simulink model "LLC_26"  (R2022b)
settings: Solver=VariableStepAuto  StartTime=0.0  StopTime=.01  RelTol=1e-3
values from neighbouring files (symbols this model uses):
  tsample_Controller = 20e-6    (= 2e-05)    [LLC_Parameter.m]
  Vref = 500    [LLC_Parameter.m]
undefined symbols (not defined in the file or in its folder): Iref
libraries: fl_lib x137, ee_lib x83, nesl_utility x63, slpidlib x7, slctrlblks x1
(part 5 of 5)

== system LLC_26/Subsystem5 ==
  Capacitor : ee_lib/Passive/Capacitor  cap_option=0  c=10e-6 F  Cvec=[1e-05, 1e-06] F  Vvec=[0, 10] V  CV_table_symmetry=1  f_vec=[1, 10] kHz  DFext_vec=[.8, 1.2]  enable_C_tol=0  C_tol=5  tol_distribution=1  nSigma=4  r=1e-6 Ohm  g=0 1/Ohm  averaging_period=0 s  enable_operating_limits=0  operating_limit_action=2  max_working_voltage_range=[-25, 25] V  power_rating=1 W  enable_faults=0  fault_action=1  Cscale_faulted=100  R_faulted=1e-3 Ohm  G_faulted=0 1/Ohm  tau_fault=1e-3 s  enable_temporal_fault=0  t_fault=1 s  enable_behavioral_fault=0  max_permissible_voltage_range=[-100, 100] V  t_fail_on_voltage=1 s  i_specify=off  i_priority=None  i=0 A  i_nominal_specify=off  i_nominal_unit=A  i_nominal_value=1  v_specify=off  v_priority=None  v=0 V  v_nominal_specify=off  v_nominal_unit=V  v_nominal_value=1  vc_specify=off  vc_priority=High  vc=0 V  vc_nominal_specify=off  vc_nominal_unit=V  vc_nominal_value=1
  Da{34..35,43..44} (4 alike) : ee_lib/Semiconductors & Converters/Diode  ModelType=ee.enum.diode.modelType.pwl  TableType=ee.enum.diode.tableType.IfMat  IfMat=[.07, .12, .19, 1.75, 4.24, 7.32, 11.2; .16, .3, .72, 2.14, 4.02, 6.35, 9.12] A  VfMat=[.9, 1.15, 1.25, 1.5, 1.75, 2.17, 2.6, 2.85; .58, .68, .75, 1.1, 1.38, 1.77, 2.27, 2.7] V  TjVec=[25, 125] degC  VfVec=[.5, .7, .9, 1.3, 1.7, 2.1, 2.5] V  IfVec=[.1, .2, .5, 1, 2, 4, 7, 10] A  Vf=Vf V  Ron=Ron Ohm  Goff=1e-8 1/Ohm  prmExp=ee.enum.diode.expParam.useTwo  I12=[.0137, .545] A  V12=[.6, .7] V  RS=0 Ohm  Tmeas=25 degC  IS=1e-12 A  ec=1  I1=0.0137 A  V1=0.6 V  N_series=1  N_parallel=1  Rz=0.3 Ohm  BV=inf V  C_param=ee.enum.diode.capParam.fixed  CJ=0 pF  CJ0=5 pF  Vvec=[.1, 10, 100] V  Cvec=[3.5, 1, .4] pF  VJ=1 V  Mgrad=0.5  FC=0.5  Q_param=ee.enum.diode.recoveryParam.off  iRM=-7.15 A  iF=4 A  didt=-750 A/us  trr_factor=3  trr=115 ns  Qrr=1500 s*uA  Vr=-600 V  Ls=150 nH  Erec=0.03 J  TT=50 ns  tau=100 ns  T_param=ee.enum.diode.temperatureParam.off  Tdevice=25 degC  I1_T2=0.245 A  V1_T2=0.5 V  IS_T2=1.25e-7 A  Tmeas2=125 degC  XTI_param=ee.enum.diode.xtiParam.pn  XTI=3  EG_param=ee.enum.diode.egapParam.material_si  EG=1.11 eV  dBVdT=0 V/K  enable_faults=simscape.enum.onoff.off  fault_action=simscape.enum.assert.action.none  fault_types=ee.enum.diode.faults.open  tau_fault=1e-3 s  IfMat_faulted=[.07, .12, .19, 1.75, 4.24, 7.32, 11.2; .16, .3, .72, 2.14, 4.02, 6.35, 9.12] A  VfMat_faulted=[.9, 1.15, 1.25, 1.5, 1.75, 2.17, 2.6, 2.85; .58, .68, .75, 1.1, 1.38, 1.77, 2.27, 2.7] V  VfVec_faulted=[.5, .7, .9, 1.3, 1.7, 2.1, 2.5] V  IfVec_faulted=[.1, .2, .5, 1, 2, 4, 7, 10] A  Ropen_faulted=1000 Ohm  Gshort_faulted=1000 1/Ohm  Vf_faulted=0.6 V  Ron_faulted=0.3 Ohm  Goff_faulted=1e-8 S  I12_faulted=[.0137, .545] A  V12_faulted=[.6, .7] V  IS_faulted=1e-12 A  ec_faulted=1  I1_faulted=0.0137 A  V1_faulted=0.6 V  RS_faulted=0 Ohm  Rz_faulted=0.3 Ohm  BV_faulted=inf V  Cscale_faulted=100  enable_temporal_fault=simscape.enum.onoff.off  t_fault=inf s  enable_behavioral_fault=simscape.enum.onoff.off  max_permissible_voltage=inf V  n_fail_on_voltage=1  max_permissible_current=inf A  t_fail_on_current=1 s  max_permissible_dVdt=inf V/s  enable_fault_input=simscape.enum.onoff.off  i_specify=off  i_priority=None  i=0 A  i_nominal_specify=off  i_nominal_unit=A  i_nominal_value=1  v_specify=off  v_priority=None  v=0 V  v_nominal_specify=off  v_nominal_unit=V  v_nominal_value=1  v_capacitor_specify=off  v_capacitor_priority=None  v_capacitor=0 V  v_capacitor_nominal_specify=off  v_capacitor_nominal_unit=V  v_capacitor_nominal_value=1  i_diode_specify=off  i_diode_priority=None  i_diode=0 A  i_diode_nominal_specify=off  i_diode_nominal_unit=A  i_diode_nominal_value=1  v_diode_specify=off  v_diode_priority=None  v_diode=0 V  v_diode_nominal_specify=off  v_diode_nominal_unit=V  v_diode_nominal_value=1  i_capacitor_specify=off  i_capacitor_priority=None  i_capacitor=0 A  i_capacitor_nominal_specify=off  i_capacitor_nominal_unit=A  i_capacitor_nominal_value=1  power_dissipated_specify=off  power_dissipated_priority=None  power_dissipated=0 W  power_dissipated_nominal_specify=off  power_dissipated_nominal_unit=W  power_dissipated_nominal_value=1  fidelity_level=ee.enum.diode.fidelity.includeChargeDyn  rec_loss_model=ee.enum.diode.reverseRecoveryModel.fixed  ErecVal=0 J  ErecMat=zeros(2, 3) J  TjrecVec=[298.15, 398.15] K  IfrecVec=[.1, 1, 10] A  VrecVal=10 V  tFilter=1 / 1000 / 100 s  max_permissible_temperature=inf K  t_fail_on_temperature=1 s  thermal_network_parameterization=ee.enum.thermalNetworkTopology.junctionCase  Rth=[0, 10] K/W  Rth_Cauer=[1, 3, 10] K/W  Rth_Foster=[4, 6] K/W  thermal_mass_parameterization=ee.enum.thermalNetwork.timeconstant  thermal_mass=[0, 1] J/K  thermal_mass_Cauer=[.1, .3, 1] J/K  thermal_mass_Foster=[1.5, 3] J/K  thermal_time_constant=[0, 10] s  thermal_time_constant_Cauer=[1, 3, 10] s  thermal_time_constant_Foster=[6, 18] s  thermal_mass_initial_temperatures=[25, 25] degC  thermal_mass_initial_temperatures_Cauer=[25, 25, 25] degC  junction_thermal_mass=0.01 J/K  Tvec_initial_Foster=[25, 25, 25, 25] degC  no_thermal_network=0  junction_temperature_specify=off  junction_temperature_priority=None  junction_temperature=25 degC  junction_temperature_nominal_specify=off  junction_temperature_nominal_unit=degC  junction_temperature_nominal_value=1
  Ph : PMIOPort  Side=Left
  N : PMIOPort  Port=2  Side=Left
  DC+ : PMIOPort  Port=3  Side=Right
  DC- : PMIOPort  Port=4  Side=Right
  connections:
  Da35/RConn1 -- Da43/LConn1 -- N/RConn1
  Da34/RConn1 -- Da44/LConn1 -- Ph/RConn1
  Da34/LConn1 -- Capacitor/RConn1 -- DC-/RConn1 -- Da35/LConn1
  DC+/RConn1 -- Da44/RConn1 -- Da43/RConn1 -- Capacitor/LConn1

== system LLC_26/Subsystem6 ==
  Capacitor : ee_lib/Passive/Capacitor  cap_option=0  c=10e-6 F  Cvec=[1e-05, 1e-06] F  Vvec=[0, 10] V  CV_table_symmetry=1  f_vec=[1, 10] kHz  DFext_vec=[.8, 1.2]  enable_C_tol=0  C_tol=5  tol_distribution=1  nSigma=4  r=1e-6 Ohm  g=0 1/Ohm  averaging_period=0 s  enable_operating_limits=0  operating_limit_action=2  max_working_voltage_range=[-25, 25] V  power_rating=1 W  enable_faults=0  fault_action=1  Cscale_faulted=100  R_faulted=1e-3 Ohm  G_faulted=0 1/Ohm  tau_fault=1e-3 s  enable_temporal_fault=0  t_fault=1 s  enable_behavioral_fault=0  max_permissible_voltage_range=[-100, 100] V  t_fail_on_voltage=1 s  i_specify=off  i_priority=None  i=0 A  i_nominal_specify=off  i_nominal_unit=A  i_nominal_value=1  v_specify=off  v_priority=None  v=0 V  v_nominal_specify=off  v_nominal_unit=V  v_nominal_value=1  vc_specify=off  vc_priority=High  vc=0 V  vc_nominal_specify=off  vc_nominal_unit=V  vc_nominal_value=1
  Capacitor1 : ee_lib/Passive/Capacitor  cap_option=0  c=10e-6 F  Cvec=[1e-05, 1e-06] F  Vvec=[0, 10] V  CV_table_symmetry=1  f_vec=[1, 10] kHz  DFext_vec=[.8, 1.2]  enable_C_tol=0  C_tol=5  tol_distribution=1  nSigma=4  r=1e-6 Ohm  g=0 1/Ohm  averaging_period=0 s  enable_operating_limits=0  operating_limit_action=2  max_working_voltage_range=[-25, 25] V  power_rating=1 W  enable_faults=0  fault_action=1  Cscale_faulted=100  R_faulted=1e-3 Ohm  G_faulted=0 1/Ohm  tau_fault=1e-3 s  enable_temporal_fault=0  t_fault=1 s  enable_behavioral_fault=0  max_permissible_voltage_range=[-100, 100] V  t_fail_on_voltage=1 s  i_specify=off  i_priority=None  i=0 A  i_nominal_specify=off  i_nominal_unit=A  i_nominal_value=1  v_specify=off  v_priority=None  v=0 V  v_nominal_specify=off  v_nominal_unit=V  v_nominal_value=1  vc_specify=off  vc_priority=High  vc=0 V  vc_nominal_specify=off  vc_nominal_unit=V  vc_nominal_value=1
  Da{34..35,43..44} (4 alike) : ee_lib/Semiconductors & Converters/Diode  ModelType=ee.enum.diode.modelType.pwl  TableType=ee.enum.diode.tableType.IfMat  IfMat=[.07, .12, .19, 1.75, 4.24, 7.32, 11.2; .16, .3, .72, 2.14, 4.02, 6.35, 9.12] A  VfMat=[.9, 1.15, 1.25, 1.5, 1.75, 2.17, 2.6, 2.85; .58, .68, .75, 1.1, 1.38, 1.77, 2.27, 2.7] V  TjVec=[25, 125] degC  VfVec=[.5, .7, .9, 1.3, 1.7, 2.1, 2.5] V  IfVec=[.1, .2, .5, 1, 2, 4, 7, 10] A  Vf=Vf V  Ron=Ron Ohm  Goff=1e-8 1/Ohm  prmExp=ee.enum.diode.expParam.useTwo  I12=[.0137, .545] A  V12=[.6, .7] V  RS=0 Ohm  Tmeas=25 degC  IS=1e-12 A  ec=1  I1=0.0137 A  V1=0.6 V  N_series=1  N_parallel=1  Rz=0.3 Ohm  BV=inf V  C_param=ee.enum.diode.capParam.fixed  CJ=0 pF  CJ0=5 pF  Vvec=[.1, 10, 100] V  Cvec=[3.5, 1, .4] pF  VJ=1 V  Mgrad=0.5  FC=0.5  Q_param=ee.enum.diode.recoveryParam.off  iRM=-7.15 A  iF=4 A  didt=-750 A/us  trr_factor=3  trr=115 ns  Qrr=1500 s*uA  Vr=-600 V  Ls=150 nH  Erec=0.03 J  TT=50 ns  tau=100 ns  T_param=ee.enum.diode.temperatureParam.off  Tdevice=25 degC  I1_T2=0.245 A  V1_T2=0.5 V  IS_T2=1.25e-7 A  Tmeas2=125 degC  XTI_param=ee.enum.diode.xtiParam.pn  XTI=3  EG_param=ee.enum.diode.egapParam.material_si  EG=1.11 eV  dBVdT=0 V/K  enable_faults=simscape.enum.onoff.off  fault_action=simscape.enum.assert.action.none  fault_types=ee.enum.diode.faults.open  tau_fault=1e-3 s  IfMat_faulted=[.07, .12, .19, 1.75, 4.24, 7.32, 11.2; .16, .3, .72, 2.14, 4.02, 6.35, 9.12] A  VfMat_faulted=[.9, 1.15, 1.25, 1.5, 1.75, 2.17, 2.6, 2.85; .58, .68, .75, 1.1, 1.38, 1.77, 2.27, 2.7] V  VfVec_faulted=[.5, .7, .9, 1.3, 1.7, 2.1, 2.5] V  IfVec_faulted=[.1, .2, .5, 1, 2, 4, 7, 10] A  Ropen_faulted=1000 Ohm  Gshort_faulted=1000 1/Ohm  Vf_faulted=0.6 V  Ron_faulted=0.3 Ohm  Goff_faulted=1e-8 S  I12_faulted=[.0137, .545] A  V12_faulted=[.6, .7] V  IS_faulted=1e-12 A  ec_faulted=1  I1_faulted=0.0137 A  V1_faulted=0.6 V  RS_faulted=0 Ohm  Rz_faulted=0.3 Ohm  BV_faulted=inf V  Cscale_faulted=100  enable_temporal_fault=simscape.enum.onoff.off  t_fault=inf s  enable_behavioral_fault=simscape.enum.onoff.off  max_permissible_voltage=inf V  n_fail_on_voltage=1  max_permissible_current=inf A  t_fail_on_current=1 s  max_permissible_dVdt=inf V/s  enable_fault_input=simscape.enum.onoff.off  i_specify=off  i_priority=None  i=0 A  i_nominal_specify=off  i_nominal_unit=A  i_nominal_value=1  v_specify=off  v_priority=None  v=0 V  v_nominal_specify=off  v_nominal_unit=V  v_nominal_value=1  v_capacitor_specify=off  v_capacitor_priority=None  v_capacitor=0 V  v_capacitor_nominal_specify=off  v_capacitor_nominal_unit=V  v_capacitor_nominal_value=1  i_diode_specify=off  i_diode_priority=None  i_diode=0 A  i_diode_nominal_specify=off  i_diode_nominal_unit=A  i_diode_nominal_value=1  v_diode_specify=off  v_diode_priority=None  v_diode=0 V  v_diode_nominal_specify=off  v_diode_nominal_unit=V  v_diode_nominal_value=1  i_capacitor_specify=off  i_capacitor_priority=None  i_capacitor=0 A  i_capacitor_nominal_specify=off  i_capacitor_nominal_unit=A  i_capacitor_nominal_value=1  power_dissipated_specify=off  power_dissipated_priority=None  power_dissipated=0 W  power_dissipated_nominal_specify=off  power_dissipated_nominal_unit=W  power_dissipated_nominal_value=1  fidelity_level=ee.enum.diode.fidelity.includeChargeDyn  rec_loss_model=ee.enum.diode.reverseRecoveryModel.fixed  ErecVal=0 J  ErecMat=zeros(2, 3) J  TjrecVec=[298.15, 398.15] K  IfrecVec=[.1, 1, 10] A  VrecVal=10 V  tFilter=1 / 1000 / 100 s  max_permissible_temperature=inf K  t_fail_on_temperature=1 s  thermal_network_parameterization=ee.enum.thermalNetworkTopology.junctionCase  Rth=[0, 10] K/W  Rth_Cauer=[1, 3, 10] K/W  Rth_Foster=[4, 6] K/W  thermal_mass_parameterization=ee.enum.thermalNetwork.timeconstant  thermal_mass=[0, 1] J/K  thermal_mass_Cauer=[.1, .3, 1] J/K  thermal_mass_Foster=[1.5, 3] J/K  thermal_time_constant=[0, 10] s  thermal_time_constant_Cauer=[1, 3, 10] s  thermal_time_constant_Foster=[6, 18] s  thermal_mass_initial_temperatures=[25, 25] degC  thermal_mass_initial_temperatures_Cauer=[25, 25, 25] degC  junction_thermal_mass=0.01 J/K  Tvec_initial_Foster=[25, 25, 25, 25] degC  no_thermal_network=0  junction_temperature_specify=off  junction_temperature_priority=None  junction_temperature=25 degC  junction_temperature_nominal_specify=off  junction_temperature_nominal_unit=degC  junction_temperature_nominal_value=1
  Ph : PMIOPort  Side=Left
  N : PMIOPort  Port=2  Side=Left
  DC+ : PMIOPort  Port=3  Side=Right
  DC- : PMIOPort  Port=4  Side=Right
  connections:
  Da35/RConn1 -- Da43/LConn1 -- N/RConn1
  Da34/RConn1 -- Da44/LConn1 -- Ph/RConn1
  Da34/LConn1 -- Capacitor/RConn1 -- DC-/RConn1 -- Capacitor1/RConn1 -- Da35/LConn1
  DC+/RConn1 -- Capacitor1/LConn1 -- Da44/RConn1 -- Da43/RConn1 -- Capacitor/LConn1

== system LLC_26/Subsystem7 ==
  Capacitor : ee_lib/Passive/Capacitor  cap_option=0  c=10e-6 F  Cvec=[1e-05, 1e-06] F  Vvec=[0, 10] V  CV_table_symmetry=1  f_vec=[1, 10] kHz  DFext_vec=[.8, 1.2]  enable_C_tol=0  C_tol=5  tol_distribution=1  nSigma=4  r=1e-6 Ohm  g=0 1/Ohm  averaging_period=0 s  enable_operating_limits=0  operating_limit_action=2  max_working_voltage_range=[-25, 25] V  power_rating=1 W  enable_faults=0  fault_action=1  Cscale_faulted=100  R_faulted=1e-3 Ohm  G_faulted=0 1/Ohm  tau_fault=1e-3 s  enable_temporal_fault=0  t_fault=1 s  enable_behavioral_fault=0  max_permissible_voltage_range=[-100, 100] V  t_fail_on_voltage=1 s  i_specify=off  i_priority=None  i=0 A  i_nominal_specify=off  i_nominal_unit=A  i_nominal_value=1  v_specify=off  v_priority=None  v=0 V  v_nominal_specify=off  v_nominal_unit=V  v_nominal_value=1  vc_specify=off  vc_priority=High  vc=0 V  vc_nominal_specify=off  vc_nominal_unit=V  vc_nominal_value=1
  Da{34..35,43..44} (4 alike) : ee_lib/Semiconductors & Converters/Diode  ModelType=ee.enum.diode.modelType.pwl  TableType=ee.enum.diode.tableType.IfMat  IfMat=[.07, .12, .19, 1.75, 4.24, 7.32, 11.2; .16, .3, .72, 2.14, 4.02, 6.35, 9.12] A  VfMat=[.9, 1.15, 1.25, 1.5, 1.75, 2.17, 2.6, 2.85; .58, .68, .75, 1.1, 1.38, 1.77, 2.27, 2.7] V  TjVec=[25, 125] degC  VfVec=[.5, .7, .9, 1.3, 1.7, 2.1, 2.5] V  IfVec=[.1, .2, .5, 1, 2, 4, 7, 10] A  Vf=Vf V  Ron=Ron Ohm  Goff=1e-8 1/Ohm  prmExp=ee.enum.diode.expParam.useTwo  I12=[.0137, .545] A  V12=[.6, .7] V  RS=0 Ohm  Tmeas=25 degC  IS=1e-12 A  ec=1  I1=0.0137 A  V1=0.6 V  N_series=1  N_parallel=1  Rz=0.3 Ohm  BV=inf V  C_param=ee.enum.diode.capParam.fixed  CJ=0 pF  CJ0=5 pF  Vvec=[.1, 10, 100] V  Cvec=[3.5, 1, .4] pF  VJ=1 V  Mgrad=0.5  FC=0.5  Q_param=ee.enum.diode.recoveryParam.off  iRM=-7.15 A  iF=4 A  didt=-750 A/us  trr_factor=3  trr=115 ns  Qrr=1500 s*uA  Vr=-600 V  Ls=150 nH  Erec=0.03 J  TT=50 ns  tau=100 ns  T_param=ee.enum.diode.temperatureParam.off  Tdevice=25 degC  I1_T2=0.245 A  V1_T2=0.5 V  IS_T2=1.25e-7 A  Tmeas2=125 degC  XTI_param=ee.enum.diode.xtiParam.pn  XTI=3  EG_param=ee.enum.diode.egapParam.material_si  EG=1.11 eV  dBVdT=0 V/K  enable_faults=simscape.enum.onoff.off  fault_action=simscape.enum.assert.action.none  fault_types=ee.enum.diode.faults.open  tau_fault=1e-3 s  IfMat_faulted=[.07, .12, .19, 1.75, 4.24, 7.32, 11.2; .16, .3, .72, 2.14, 4.02, 6.35, 9.12] A  VfMat_faulted=[.9, 1.15, 1.25, 1.5, 1.75, 2.17, 2.6, 2.85; .58, .68, .75, 1.1, 1.38, 1.77, 2.27, 2.7] V  VfVec_faulted=[.5, .7, .9, 1.3, 1.7, 2.1, 2.5] V  IfVec_faulted=[.1, .2, .5, 1, 2, 4, 7, 10] A  Ropen_faulted=1000 Ohm  Gshort_faulted=1000 1/Ohm  Vf_faulted=0.6 V  Ron_faulted=0.3 Ohm  Goff_faulted=1e-8 S  I12_faulted=[.0137, .545] A  V12_faulted=[.6, .7] V  IS_faulted=1e-12 A  ec_faulted=1  I1_faulted=0.0137 A  V1_faulted=0.6 V  RS_faulted=0 Ohm  Rz_faulted=0.3 Ohm  BV_faulted=inf V  Cscale_faulted=100  enable_temporal_fault=simscape.enum.onoff.off  t_fault=inf s  enable_behavioral_fault=simscape.enum.onoff.off  max_permissible_voltage=inf V  n_fail_on_voltage=1  max_permissible_current=inf A  t_fail_on_current=1 s  max_permissible_dVdt=inf V/s  enable_fault_input=simscape.enum.onoff.off  i_specify=off  i_priority=None  i=0 A  i_nominal_specify=off  i_nominal_unit=A  i_nominal_value=1  v_specify=off  v_priority=None  v=0 V  v_nominal_specify=off  v_nominal_unit=V  v_nominal_value=1  v_capacitor_specify=off  v_capacitor_priority=None  v_capacitor=0 V  v_capacitor_nominal_specify=off  v_capacitor_nominal_unit=V  v_capacitor_nominal_value=1  i_diode_specify=off  i_diode_priority=None  i_diode=0 A  i_diode_nominal_specify=off  i_diode_nominal_unit=A  i_diode_nominal_value=1  v_diode_specify=off  v_diode_priority=None  v_diode=0 V  v_diode_nominal_specify=off  v_diode_nominal_unit=V  v_diode_nominal_value=1  i_capacitor_specify=off  i_capacitor_priority=None  i_capacitor=0 A  i_capacitor_nominal_specify=off  i_capacitor_nominal_unit=A  i_capacitor_nominal_value=1  power_dissipated_specify=off  power_dissipated_priority=None  power_dissipated=0 W  power_dissipated_nominal_specify=off  power_dissipated_nominal_unit=W  power_dissipated_nominal_value=1  fidelity_level=ee.enum.diode.fidelity.includeChargeDyn  rec_loss_model=ee.enum.diode.reverseRecoveryModel.fixed  ErecVal=0 J  ErecMat=zeros(2, 3) J  TjrecVec=[298.15, 398.15] K  IfrecVec=[.1, 1, 10] A  VrecVal=10 V  tFilter=1 / 1000 / 100 s  max_permissible_temperature=inf K  t_fail_on_temperature=1 s  thermal_network_parameterization=ee.enum.thermalNetworkTopology.junctionCase  Rth=[0, 10] K/W  Rth_Cauer=[1, 3, 10] K/W  Rth_Foster=[4, 6] K/W  thermal_mass_parameterization=ee.enum.thermalNetwork.timeconstant  thermal_mass=[0, 1] J/K  thermal_mass_Cauer=[.1, .3, 1] J/K  thermal_mass_Foster=[1.5, 3] J/K  thermal_time_constant=[0, 10] s  thermal_time_constant_Cauer=[1, 3, 10] s  thermal_time_constant_Foster=[6, 18] s  thermal_mass_initial_temperatures=[25, 25] degC  thermal_mass_initial_temperatures_Cauer=[25, 25, 25] degC  junction_thermal_mass=0.01 J/K  Tvec_initial_Foster=[25, 25, 25, 25] degC  no_thermal_network=0  junction_temperature_specify=off  junction_temperature_priority=None  junction_temperature=25 degC  junction_temperature_nominal_specify=off  junction_temperature_nominal_unit=degC  junction_temperature_nominal_value=1
  Ph : PMIOPort  Side=Left
  N : PMIOPort  Port=2  Side=Left
  DC+ : PMIOPort  Port=3  Side=Right
  DC- : PMIOPort  Port=4  Side=Right
  connections:
  Da35/RConn1 -- Da43/LConn1 -- N/RConn1
  Da34/RConn1 -- Da44/LConn1 -- Ph/RConn1
  Da34/LConn1 -- Capacitor/RConn1 -- DC-/RConn1 -- Da35/LConn1
  DC+/RConn1 -- Da44/RConn1 -- Da43/RConn1 -- Capacitor/LConn1

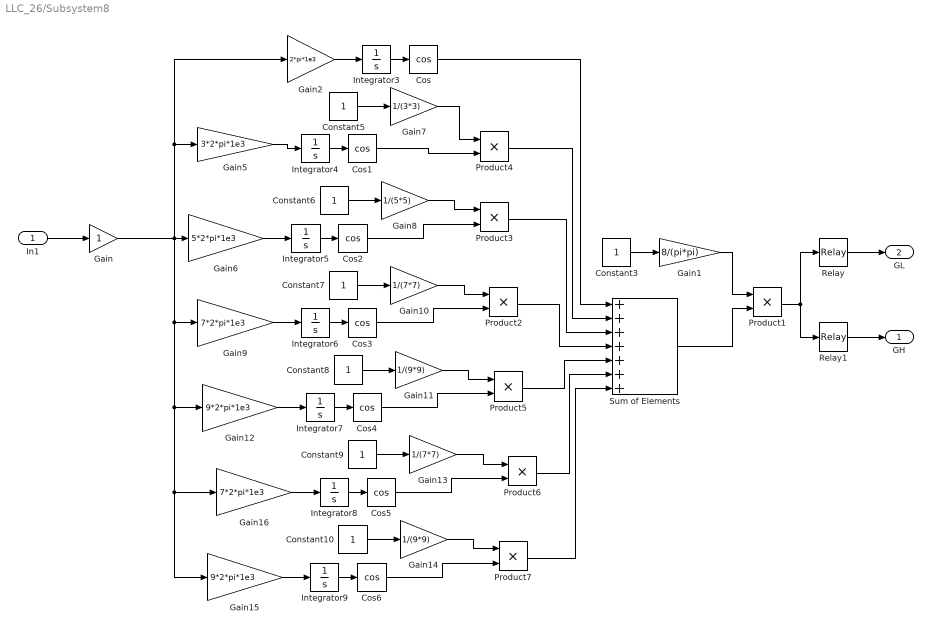
== system LLC_26/Subsystem8 ==
  In1 : Inport
  Constant{3,5..10} (7 alike) : Constant
  Cos{,1..6} (7 alike) : Trigonometry  Operator=cos
  Gain : Gain
  Gain1 : Gain  Gain=8/(pi*pi)
  Gain10 : Gain  Gain=1/(7*7)
  Gain11 : Gain  Gain=1/(9*9)
  Gain12 : Gain  Gain=9*2*pi*1e3
  Gain13 : Gain  Gain=1/(7*7)
  Gain14 : Gain  Gain=1/(9*9)
  Gain15 : Gain  Gain=9*2*pi*1e3
  Gain16 : Gain  Gain=7*2*pi*1e3
  Gain2 : Gain  Gain=2*pi*1e3
  Gain5 : Gain  Gain=3*2*pi*1e3
  Gain6 : Gain  Gain=5*2*pi*1e3
  Gain7 : Gain  Gain=1/(3*3)
  Gain8 : Gain  Gain=1/(5*5)
  Gain9 : Gain  Gain=7*2*pi*1e3
  Integrator{3..9} (7 alike) : Integrator
  Product{1..7} (7 alike) : Product
  Relay : Relay  OnSwitchValue=0.15  OffSwitchValue=-0.0001
  Relay1 : Relay  OnSwitchValue=0.0001  OffSwitchValue=-0.15  OnOutputValue=0  OffOutputValue=1
  Sum of Elements : Sum  Inputs=+++++++
  GH : Outport
  GL : Outport  Port=2
  wires:
  Product7/1 -> Sum of Elements/7
  Product5/1 -> Sum of Elements/5
  Constant5/1 -> Gain7/1
  Gain11/1 -> Product5/1
  Integrator7/1 -> Cos4/1
  Gain9/1 -> Integrator6/1
  Constant6/1 -> Gain8/1
  Product1/1 -> Relay1/1, Relay/1
  Product4/1 -> Sum of Elements/2
  Gain8/1 -> Product3/1
  Constant3/1 -> Gain1/1
  Integrator3/1 -> Cos/1
  Gain10/1 -> Product2/1
  Gain2/1 -> Integrator3/1
  Gain12/1 -> Integrator7/1
  Gain16/1 -> Integrator8/1
  Cos5/1 -> Product6/2
  Cos3/1 -> Product2/2
  Product3/1 -> Sum of Elements/3
  Constant7/1 -> Gain10/1
  Gain6/1 -> Integrator5/1
  Integrator8/1 -> Cos5/1
  Integrator4/1 -> Cos1/1
  Gain5/1 -> Integrator4/1
  Cos1/1 -> Product4/2
  Gain15/1 -> Integrator9/1
  Product2/1 -> Sum of Elements/4
  Cos/1 -> Sum of Elements/1
  Constant10/1 -> Gain14/1
  Cos2/1 -> Product3/2
  Gain1/1 -> Product1/1
  Integrator6/1 -> Cos3/1
  Product6/1 -> Sum of Elements/6
  Integrator5/1 -> Cos2/1
  Integrator9/1 -> Cos6/1
  Cos6/1 -> Product7/2
  Constant9/1 -> Gain13/1
  Gain14/1 -> Product7/1
  Cos4/1 -> Product5/2
  Gain7/1 -> Product4/1
  Constant8/1 -> Gain11/1
  Sum of Elements/1 -> Product1/2
  Gain13/1 -> Product6/1
  Relay1/1 -> GH/1
  Relay/1 -> GL/1
  Gain/1 -> Gain15/1, Gain16/1, Gain12/1, Gain9/1, Gain6/1, Gain5/1, Gain2/1
  In1/1 -> Gain/1

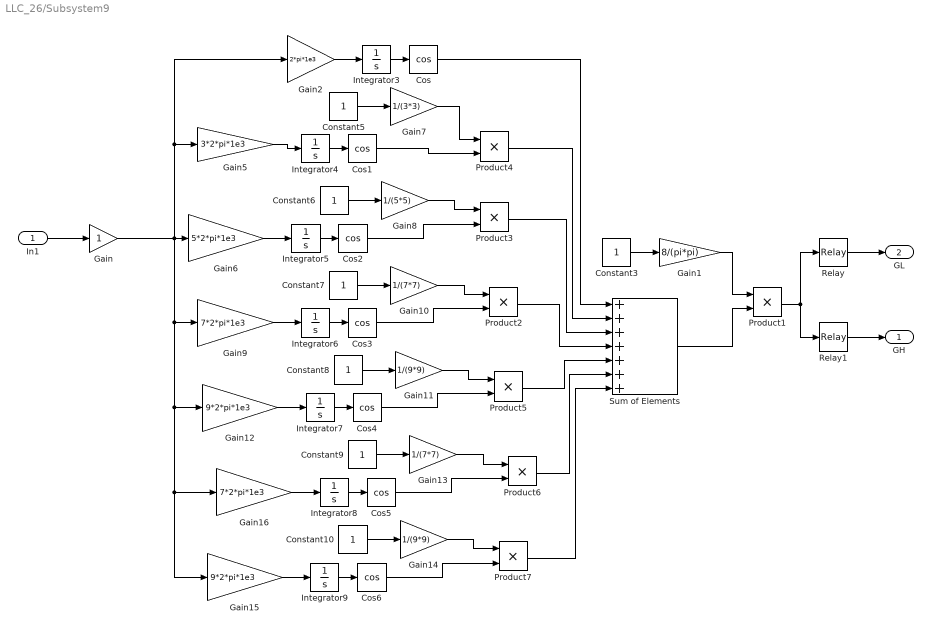
== system LLC_26/Subsystem9 ==
  In1 : Inport
  Constant{3,5..10} (7 alike) : Constant
  Cos{,1..6} (7 alike) : Trigonometry  Operator=cos
  Gain : Gain
  Gain1 : Gain  Gain=8/(pi*pi)
  Gain10 : Gain  Gain=1/(7*7)
  Gain11 : Gain  Gain=1/(9*9)
  Gain12 : Gain  Gain=9*2*pi*1e3
  Gain13 : Gain  Gain=1/(7*7)
  Gain14 : Gain  Gain=1/(9*9)
  Gain15 : Gain  Gain=9*2*pi*1e3
  Gain16 : Gain  Gain=7*2*pi*1e3
  Gain2 : Gain  Gain=2*pi*1e3
  Gain5 : Gain  Gain=3*2*pi*1e3
  Gain6 : Gain  Gain=5*2*pi*1e3
  Gain7 : Gain  Gain=1/(3*3)
  Gain8 : Gain  Gain=1/(5*5)
  Gain9 : Gain  Gain=7*2*pi*1e3
  Integrator{3..9} (7 alike) : Integrator
  Product{1..7} (7 alike) : Product
  Relay : Relay  OnSwitchValue=0.15  OffSwitchValue=-0.0001
  Relay1 : Relay  OnSwitchValue=0.0001  OffSwitchValue=-0.15  OnOutputValue=0  OffOutputValue=1
  Sum of Elements : Sum  Inputs=+++++++
  GH : Outport
  GL : Outport  Port=2
  wires:
  Product7/1 -> Sum of Elements/7
  Product5/1 -> Sum of Elements/5
  Constant5/1 -> Gain7/1
  Gain11/1 -> Product5/1
  Integrator7/1 -> Cos4/1
  Gain9/1 -> Integrator6/1
  Constant6/1 -> Gain8/1
  Product1/1 -> Relay1/1, Relay/1
  Product4/1 -> Sum of Elements/2
  Gain8/1 -> Product3/1
  Constant3/1 -> Gain1/1
  Integrator3/1 -> Cos/1
  Gain10/1 -> Product2/1
  Gain2/1 -> Integrator3/1
  Gain12/1 -> Integrator7/1
  Gain16/1 -> Integrator8/1
  Cos5/1 -> Product6/2
  Cos3/1 -> Product2/2
  Product3/1 -> Sum of Elements/3
  Constant7/1 -> Gain10/1
  Gain6/1 -> Integrator5/1
  Integrator8/1 -> Cos5/1
  Integrator4/1 -> Cos1/1
  Gain5/1 -> Integrator4/1
  Cos1/1 -> Product4/2
  Gain15/1 -> Integrator9/1
  Product2/1 -> Sum of Elements/4
  Cos/1 -> Sum of Elements/1
  Constant10/1 -> Gain14/1
  Cos2/1 -> Product3/2
  Gain1/1 -> Product1/1
  Integrator6/1 -> Cos3/1
  Product6/1 -> Sum of Elements/6
  Integrator5/1 -> Cos2/1
  Integrator9/1 -> Cos6/1
  Cos6/1 -> Product7/2
  Constant9/1 -> Gain13/1
  Gain14/1 -> Product7/1
  Cos4/1 -> Product5/2
  Gain7/1 -> Product4/1
  Constant8/1 -> Gain11/1
  Sum of Elements/1 -> Product1/2
  Gain13/1 -> Product6/1
  Relay1/1 -> GH/1
  Relay/1 -> GL/1
  Gain/1 -> Gain15/1, Gain16/1, Gain12/1, Gain9/1, Gain6/1, Gain5/1, Gain2/1
  In1/1 -> Gain/1

== system LLC_26/Control loop with Refernce from Micro chip/Update PID Gains ==
  In1 : Inport
  Trigger : TriggerPort  TriggerType=falling  VariantControl=Variant  PortDimensions=1
  Bus Selector : BusSelector  OutputSignals=P,I,D,N
  Mux : Mux
  Write PID Gains : DataStoreWrite  DataStoreName=Gains  IndexOptions=Index vector (dialog)  Indices=1  OutputSizes=1
  wires:
  In1/1 -> Bus Selector/1
  Bus Selector/1 -> Mux/1  "<P>"
  Bus Selector/2 -> Mux/2  "<I>"
  Bus Selector/3 -> Mux/3  "<D>"
  Bus Selector/4 -> Mux/4  "<N>"
  Mux/1 -> Write PID Gains/1

== system LLC_26/Subsystem12/Current Sensor Primary ==
  ERef : fl_lib/Electrical/Electrical Elements/Electrical Reference
  Ip : fl_lib/Electrical/Electrical Sensors/Current Sensor
  PS-Simulink Converter 3 : nesl_utility/PS-Simulink Converter  PhysicalDomain=network_engine_domain  SubClassName=ps_output  LeftPortType=input  RightPortType=output  PseudoPeriodic=off  Frequencies=[]  VectorFormat=1-D array  Unit=1  AffineConversion=off
  PS-Simulink Converter 5 : nesl_utility/PS-Simulink Converter  PhysicalDomain=network_engine_domain  SubClassName=ps_output  LeftPortType=input  RightPortType=output  PseudoPeriodic=off  Frequencies=[]  VectorFormat=1-D array  Unit=1  AffineConversion=off
  Vp : fl_lib/Electrical/Electrical Sensors/Voltage Sensor
  + : PMIOPort  Side=Left
  - : PMIOPort  Port=2  Side=Right
  tag scope: i11=global, v11=global
  wires:
  PS-Simulink Converter 3/1 -> [i11]  "Primary (A)"
  PS-Simulink Converter 5/1 -> [v11]  "Primary (V)"
  connections:
  Ip/RConn2 -- -/RConn1
  +/RConn1 -- Vp/LConn1 -- Ip/LConn1
  Ip/RConn1 -- PS-Simulink Converter 3/LConn1
  PS-Simulink Converter 5/LConn1 -- Vp/RConn1
  ERef/LConn1 -- Vp/RConn2

== system LLC_26/Subsystem12/Current Sensor Secondary ==
  ERef : fl_lib/Electrical/Electrical Elements/Electrical Reference
  Ip : fl_lib/Electrical/Electrical Sensors/Current Sensor
  PS-Simulink Converter 4 : nesl_utility/PS-Simulink Converter  PhysicalDomain=network_engine_domain  SubClassName=ps_output  LeftPortType=input  RightPortType=output  PseudoPeriodic=off  Frequencies=[]  VectorFormat=1-D array  Unit=1  AffineConversion=off
  PS-Simulink Converter 5 : nesl_utility/PS-Simulink Converter  PhysicalDomain=network_engine_domain  SubClassName=ps_output  LeftPortType=input  RightPortType=output  PseudoPeriodic=off  Frequencies=[]  VectorFormat=1-D array  Unit=1  AffineConversion=off
  Vp : fl_lib/Electrical/Electrical Sensors/Voltage Sensor
  + : PMIOPort  Side=Left
  - : PMIOPort  Port=2  Side=Right
  tag scope: i21=global, v21=global
  wires:
  PS-Simulink Converter 4/1 -> [i21]  "Secondary (A)"
  PS-Simulink Converter 5/1 -> [v21]  "Secondary  (V)"
  connections:
  PS-Simulink Converter 4/LConn1 -- Ip/RConn1
  +/RConn1 -- Vp/LConn1 -- Ip/LConn1
  Ip/RConn2 -- -/RConn1
  PS-Simulink Converter 5/LConn1 -- Vp/RConn1
  ERef/LConn1 -- Vp/RConn2

== system LLC_26/Subsystem12/Current Sensor Secondary1 ==
  ERef : fl_lib/Electrical/Electrical Elements/Electrical Reference
  Ip : fl_lib/Electrical/Electrical Sensors/Current Sensor
  PS-Simulink Converter 4 : nesl_utility/PS-Simulink Converter  PhysicalDomain=network_engine_domain  SubClassName=ps_output  LeftPortType=input  RightPortType=output  PseudoPeriodic=off  Frequencies=[]  VectorFormat=1-D array  Unit=1  AffineConversion=off
  PS-Simulink Converter 5 : nesl_utility/PS-Simulink Converter  PhysicalDomain=network_engine_domain  SubClassName=ps_output  LeftPortType=input  RightPortType=output  PseudoPeriodic=off  Frequencies=[]  VectorFormat=1-D array  Unit=1  AffineConversion=off
  Vp : fl_lib/Electrical/Electrical Sensors/Voltage Sensor
  + : PMIOPort  Side=Left
  - : PMIOPort  Port=2  Side=Right
  tag scope: i31=global, v31=global
  wires:
  PS-Simulink Converter 4/1 -> [i31]  "Secondary (A)"
  PS-Simulink Converter 5/1 -> [v31]  "Secondary  (V)"
  connections:
  PS-Simulink Converter 4/LConn1 -- Ip/RConn1
  +/RConn1 -- Vp/LConn1 -- Ip/LConn1
  Ip/RConn2 -- -/RConn1
  PS-Simulink Converter 5/LConn1 -- Vp/RConn1
  ERef/LConn1 -- Vp/RConn2

== system LLC_26/Subsystem13/Current Sensor Primary ==
  ERef : fl_lib/Electrical/Electrical Elements/Electrical Reference
  Ip : fl_lib/Electrical/Electrical Sensors/Current Sensor
  PS-Simulink Converter 3 : nesl_utility/PS-Simulink Converter  PhysicalDomain=network_engine_domain  SubClassName=ps_output  LeftPortType=input  RightPortType=output  PseudoPeriodic=off  Frequencies=[]  VectorFormat=1-D array  Unit=1  AffineConversion=off
  PS-Simulink Converter 5 : nesl_utility/PS-Simulink Converter  PhysicalDomain=network_engine_domain  SubClassName=ps_output  LeftPortType=input  RightPortType=output  PseudoPeriodic=off  Frequencies=[]  VectorFormat=1-D array  Unit=1  AffineConversion=off
  Vp : fl_lib/Electrical/Electrical Sensors/Voltage Sensor
  + : PMIOPort  Side=Left
  - : PMIOPort  Port=2  Side=Right
  tag scope: i12=global, v12=global
  wires:
  PS-Simulink Converter 3/1 -> [i12]  "Primary (A)"
  PS-Simulink Converter 5/1 -> [v12]  "Primary (V)"
  connections:
  Ip/RConn2 -- -/RConn1
  +/RConn1 -- Vp/LConn1 -- Ip/LConn1
  Ip/RConn1 -- PS-Simulink Converter 3/LConn1
  PS-Simulink Converter 5/LConn1 -- Vp/RConn1
  ERef/LConn1 -- Vp/RConn2

== system LLC_26/Subsystem13/Current Sensor Secondary ==
  ERef : fl_lib/Electrical/Electrical Elements/Electrical Reference
  Ip : fl_lib/Electrical/Electrical Sensors/Current Sensor
  PS-Simulink Converter 4 : nesl_utility/PS-Simulink Converter  PhysicalDomain=network_engine_domain  SubClassName=ps_output  LeftPortType=input  RightPortType=output  PseudoPeriodic=off  Frequencies=[]  VectorFormat=1-D array  Unit=1  AffineConversion=off
  PS-Simulink Converter 5 : nesl_utility/PS-Simulink Converter  PhysicalDomain=network_engine_domain  SubClassName=ps_output  LeftPortType=input  RightPortType=output  PseudoPeriodic=off  Frequencies=[]  VectorFormat=1-D array  Unit=1  AffineConversion=off
  Vp : fl_lib/Electrical/Electrical Sensors/Voltage Sensor
  + : PMIOPort  Side=Left
  - : PMIOPort  Port=2  Side=Right
  tag scope: i22=global, v22=global
  wires:
  PS-Simulink Converter 4/1 -> [i22]  "Secondary (A)"
  PS-Simulink Converter 5/1 -> [v22]  "Secondary  (V)"
  connections:
  PS-Simulink Converter 4/LConn1 -- Ip/RConn1
  +/RConn1 -- Vp/LConn1 -- Ip/LConn1
  Ip/RConn2 -- -/RConn1
  PS-Simulink Converter 5/LConn1 -- Vp/RConn1
  ERef/LConn1 -- Vp/RConn2

== system LLC_26/Subsystem13/Current Sensor Secondary1 ==
  ERef : fl_lib/Electrical/Electrical Elements/Electrical Reference
  Ip : fl_lib/Electrical/Electrical Sensors/Current Sensor
  PS-Simulink Converter 4 : nesl_utility/PS-Simulink Converter  PhysicalDomain=network_engine_domain  SubClassName=ps_output  LeftPortType=input  RightPortType=output  PseudoPeriodic=off  Frequencies=[]  VectorFormat=1-D array  Unit=1  AffineConversion=off
  PS-Simulink Converter 5 : nesl_utility/PS-Simulink Converter  PhysicalDomain=network_engine_domain  SubClassName=ps_output  LeftPortType=input  RightPortType=output  PseudoPeriodic=off  Frequencies=[]  VectorFormat=1-D array  Unit=1  AffineConversion=off
  Vp : fl_lib/Electrical/Electrical Sensors/Voltage Sensor
  + : PMIOPort  Side=Left
  - : PMIOPort  Port=2  Side=Right
  tag scope: i32=global, v32=global
  wires:
  PS-Simulink Converter 4/1 -> [i32]  "Secondary (A)"
  PS-Simulink Converter 5/1 -> [v32]  "Secondary  (V)"
  connections:
  PS-Simulink Converter 4/LConn1 -- Ip/RConn1
  +/RConn1 -- Vp/LConn1 -- Ip/LConn1
  Ip/RConn2 -- -/RConn1
  PS-Simulink Converter 5/LConn1 -- Vp/RConn1
  ERef/LConn1 -- Vp/RConn2

== system LLC_26/Subsystem14/Current Sensor Primary ==
  ERef : fl_lib/Electrical/Electrical Elements/Electrical Reference
  Ip : fl_lib/Electrical/Electrical Sensors/Current Sensor
  PS-Simulink Converter 3 : nesl_utility/PS-Simulink Converter  PhysicalDomain=network_engine_domain  SubClassName=ps_output  LeftPortType=input  RightPortType=output  PseudoPeriodic=off  Frequencies=[]  VectorFormat=1-D array  Unit=1  AffineConversion=off
  PS-Simulink Converter 5 : nesl_utility/PS-Simulink Converter  PhysicalDomain=network_engine_domain  SubClassName=ps_output  LeftPortType=input  RightPortType=output  PseudoPeriodic=off  Frequencies=[]  VectorFormat=1-D array  Unit=1  AffineConversion=off
  Vp : fl_lib/Electrical/Electrical Sensors/Voltage Sensor
  + : PMIOPort  Side=Left
  - : PMIOPort  Port=2  Side=Right
  tag scope: i13=global, v13=global
  wires:
  PS-Simulink Converter 3/1 -> [i13]  "Primary (A)"
  PS-Simulink Converter 5/1 -> [v13]  "Primary (V)"
  connections:
  Ip/RConn2 -- -/RConn1
  +/RConn1 -- Vp/LConn1 -- Ip/LConn1
  Ip/RConn1 -- PS-Simulink Converter 3/LConn1
  PS-Simulink Converter 5/LConn1 -- Vp/RConn1
  ERef/LConn1 -- Vp/RConn2

== system LLC_26/Subsystem14/Current Sensor Secondary ==
  ERef : fl_lib/Electrical/Electrical Elements/Electrical Reference
  Ip : fl_lib/Electrical/Electrical Sensors/Current Sensor
  PS-Simulink Converter 4 : nesl_utility/PS-Simulink Converter  PhysicalDomain=network_engine_domain  SubClassName=ps_output  LeftPortType=input  RightPortType=output  PseudoPeriodic=off  Frequencies=[]  VectorFormat=1-D array  Unit=1  AffineConversion=off
  PS-Simulink Converter 5 : nesl_utility/PS-Simulink Converter  PhysicalDomain=network_engine_domain  SubClassName=ps_output  LeftPortType=input  RightPortType=output  PseudoPeriodic=off  Frequencies=[]  VectorFormat=1-D array  Unit=1  AffineConversion=off
  Vp : fl_lib/Electrical/Electrical Sensors/Voltage Sensor
  + : PMIOPort  Side=Left
  - : PMIOPort  Port=2  Side=Right
  tag scope: i23=global, v23=global
  wires:
  PS-Simulink Converter 4/1 -> [i23]  "Secondary (A)"
  PS-Simulink Converter 5/1 -> [v23]  "Secondary  (V)"
  connections:
  PS-Simulink Converter 4/LConn1 -- Ip/RConn1
  +/RConn1 -- Vp/LConn1 -- Ip/LConn1
  Ip/RConn2 -- -/RConn1
  PS-Simulink Converter 5/LConn1 -- Vp/RConn1
  ERef/LConn1 -- Vp/RConn2

== system LLC_26/Subsystem14/Current Sensor Secondary1 ==
  ERef : fl_lib/Electrical/Electrical Elements/Electrical Reference
  Ip : fl_lib/Electrical/Electrical Sensors/Current Sensor
  PS-Simulink Converter 4 : nesl_utility/PS-Simulink Converter  PhysicalDomain=network_engine_domain  SubClassName=ps_output  LeftPortType=input  RightPortType=output  PseudoPeriodic=off  Frequencies=[]  VectorFormat=1-D array  Unit=1  AffineConversion=off
  PS-Simulink Converter 5 : nesl_utility/PS-Simulink Converter  PhysicalDomain=network_engine_domain  SubClassName=ps_output  LeftPortType=input  RightPortType=output  PseudoPeriodic=off  Frequencies=[]  VectorFormat=1-D array  Unit=1  AffineConversion=off
  Vp : fl_lib/Electrical/Electrical Sensors/Voltage Sensor
  + : PMIOPort  Side=Left
  - : PMIOPort  Port=2  Side=Right
  tag scope: i33=global, v33=global
  wires:
  PS-Simulink Converter 4/1 -> [i33]  "Secondary (A)"
  PS-Simulink Converter 5/1 -> [v33]  "Secondary  (V)"
  connections:
  PS-Simulink Converter 4/LConn1 -- Ip/RConn1
  +/RConn1 -- Vp/LConn1 -- Ip/LConn1
  Ip/RConn2 -- -/RConn1
  PS-Simulink Converter 5/LConn1 -- Vp/RConn1
  ERef/LConn1 -- Vp/RConn2

== system LLC_26/Subsystem15/Current Sensor Primary ==
  ERef : fl_lib/Electrical/Electrical Elements/Electrical Reference
  Ip : fl_lib/Electrical/Electrical Sensors/Current Sensor
  PS-Simulink Converter 3 : nesl_utility/PS-Simulink Converter  PhysicalDomain=network_engine_domain  SubClassName=ps_output  LeftPortType=input  RightPortType=output  PseudoPeriodic=off  Frequencies=[]  VectorFormat=1-D array  Unit=1  AffineConversion=off
  PS-Simulink Converter 5 : nesl_utility/PS-Simulink Converter  PhysicalDomain=network_engine_domain  SubClassName=ps_output  LeftPortType=input  RightPortType=output  PseudoPeriodic=off  Frequencies=[]  VectorFormat=1-D array  Unit=1  AffineConversion=off
  Vp : fl_lib/Electrical/Electrical Sensors/Voltage Sensor
  + : PMIOPort  Side=Left
  - : PMIOPort  Port=2  Side=Right
  tag scope: i14=global, v14=global
  wires:
  PS-Simulink Converter 3/1 -> [i14]  "Primary (A)"
  PS-Simulink Converter 5/1 -> [v14]  "Primary (V)"
  connections:
  Ip/RConn2 -- -/RConn1
  +/RConn1 -- Vp/LConn1 -- Ip/LConn1
  Ip/RConn1 -- PS-Simulink Converter 3/LConn1
  PS-Simulink Converter 5/LConn1 -- Vp/RConn1
  ERef/LConn1 -- Vp/RConn2

== system LLC_26/Subsystem15/Current Sensor Secondary ==
  ERef : fl_lib/Electrical/Electrical Elements/Electrical Reference
  Ip : fl_lib/Electrical/Electrical Sensors/Current Sensor
  PS-Simulink Converter 4 : nesl_utility/PS-Simulink Converter  PhysicalDomain=network_engine_domain  SubClassName=ps_output  LeftPortType=input  RightPortType=output  PseudoPeriodic=off  Frequencies=[]  VectorFormat=1-D array  Unit=1  AffineConversion=off
  PS-Simulink Converter 5 : nesl_utility/PS-Simulink Converter  PhysicalDomain=network_engine_domain  SubClassName=ps_output  LeftPortType=input  RightPortType=output  PseudoPeriodic=off  Frequencies=[]  VectorFormat=1-D array  Unit=1  AffineConversion=off
  Vp : fl_lib/Electrical/Electrical Sensors/Voltage Sensor
  + : PMIOPort  Side=Left
  - : PMIOPort  Port=2  Side=Right
  tag scope: i24=global, v24=global
  wires:
  PS-Simulink Converter 4/1 -> [i24]  "Secondary (A)"
  PS-Simulink Converter 5/1 -> [v24]  "Secondary  (V)"
  connections:
  PS-Simulink Converter 4/LConn1 -- Ip/RConn1
  +/RConn1 -- Vp/LConn1 -- Ip/LConn1
  Ip/RConn2 -- -/RConn1
  PS-Simulink Converter 5/LConn1 -- Vp/RConn1
  ERef/LConn1 -- Vp/RConn2

== system LLC_26/Subsystem15/Current Sensor Secondary1 ==
  ERef : fl_lib/Electrical/Electrical Elements/Electrical Reference
  Ip : fl_lib/Electrical/Electrical Sensors/Current Sensor
  PS-Simulink Converter 4 : nesl_utility/PS-Simulink Converter  PhysicalDomain=network_engine_domain  SubClassName=ps_output  LeftPortType=input  RightPortType=output  PseudoPeriodic=off  Frequencies=[]  VectorFormat=1-D array  Unit=1  AffineConversion=off
  PS-Simulink Converter 5 : nesl_utility/PS-Simulink Converter  PhysicalDomain=network_engine_domain  SubClassName=ps_output  LeftPortType=input  RightPortType=output  PseudoPeriodic=off  Frequencies=[]  VectorFormat=1-D array  Unit=1  AffineConversion=off
  Vp : fl_lib/Electrical/Electrical Sensors/Voltage Sensor
  + : PMIOPort  Side=Left
  - : PMIOPort  Port=2  Side=Right
  tag scope: i34=global, v34=global
  wires:
  PS-Simulink Converter 4/1 -> [i34]  "Secondary (A)"
  PS-Simulink Converter 5/1 -> [v34]  "Secondary  (V)"
  connections:
  PS-Simulink Converter 4/LConn1 -- Ip/RConn1
  +/RConn1 -- Vp/LConn1 -- Ip/LConn1
  Ip/RConn2 -- -/RConn1
  PS-Simulink Converter 5/LConn1 -- Vp/RConn1
  ERef/LConn1 -- Vp/RConn2

== matlab function LLC_26/PARALLEL(-)/MATLAB Function ==
  data: mode input; y output
function y = fcn(mode)
if mode=="Parallel"
    y=5;
else
    y=0;
end

== matlab function LLC_26/PARALLEL(+)/MATLAB Function ==
  data: mode input; y output
function y = fcn(mode)
if mode=="Parallel"
    y=5;
else
    y=0;
end

== matlab function LLC_26/SERIES/MATLAB Function ==
  data: mode input; y output
function y = fcn(mode)
if mode=="Series"
    y=5;
else
    y=0;
end
